simulink model "PLCPong"  (R2020a)
settings: Solver=VariableStepAuto  StartTime=0.0  StopTime=inf  FixedStep=0.05  RelTol=1e-3
libraries: library_plc2simulink x13
settings Model: EnablePacing=on  Creator=Moritz  LastModifiedBy=Moritz

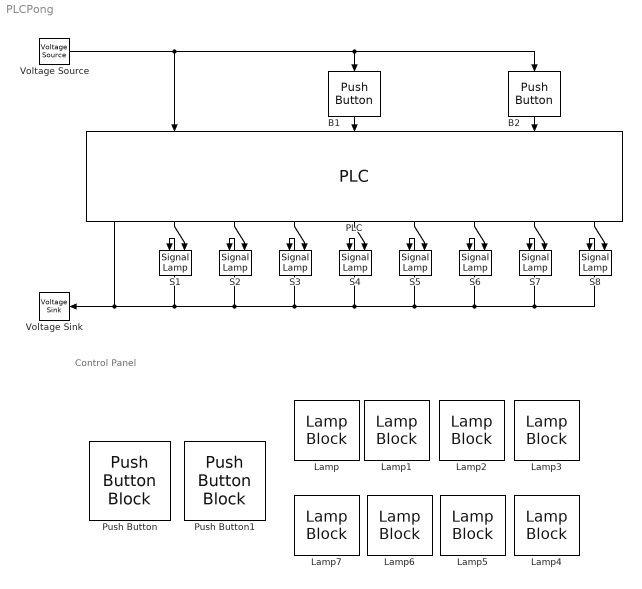
== system PLCPong ==
  note: Control Panel
  B1 : library_plc2simulink/Push Button  deactTime=0.3  StateOn=0
      settings: SourceProductName=PLC2Simulink
  B2 : library_plc2simulink/Push Button  deactTime=0.3  StateOn=0
      settings: SourceProductName=PLC2Simulink
  Lamp : LampBlock  Tag=S1  LabelPosition=Hide
      settings: AttributesFormatString=S1
  Lamp{1..7} (7 alike) : LampBlock  LabelPosition=Hide
      Lamp1 settings: AttributesFormatString=S2
      Lamp2 settings: AttributesFormatString=S3
      Lamp3 settings: AttributesFormatString=S4
      Lamp4 settings: AttributesFormatString=S5
      Lamp5 settings: AttributesFormatString=S6
      Lamp6 settings: AttributesFormatString=S7
      Lamp7 settings: AttributesFormatString=S8
  PLC : library_plc2simulink/PLC  instanceName=PLC1  numInputs=2  numOutputs=8  timeStep=0.05  externalSupplyVoltage=on
      settings: SourceProductName=PLC2Simulink
  Push Button : PushButtonBlock  ButtonText=B1
  Push Button1 : PushButtonBlock  ButtonText=B2
      settings: AttributesFormatString=B2
  S{1..8} (8 alike) : library_plc2simulink/Signal Lamp  Value=off  updateTime=0.1  colorOn=[0.2,1,0.2]  colorOff=[1,1,1]
      settings: SourceProductName=PLC2Simulink
  Voltage Sink : library_plc2simulink/Voltage Sink
      settings: SourceProductName=PLC2Simulink
  Voltage Source : library_plc2simulink/Voltage Source  voltage=24
      settings: SourceProductName=PLC2Simulink
  wires:
  Voltage Source/1 -> PLC/1, B2/1, B1/1
  PLC/1 -> Voltage Sink/1, S8/2, S7/2, S6/2, S5/2, S4/2, S3/2, S2/2, S1/2
  B1/1 -> PLC/2
  B2/1 -> PLC/3
  PLC/2 -> S1/1
  PLC/3 -> S2/1
  PLC/4 -> S3/1
  PLC/5 -> S4/1
  PLC/6 -> S5/1
  PLC/7 -> S6/1
  PLC/8 -> S7/1
  PLC/9 -> S8/1
